simulink model "testBallLQG"  (R2019b)
settings: Solver=VariableStepAuto  StartTime=0.0  StopTime=10.0  RelTol=1e-3
values from neighbouring files (symbols this model uses):
  Ab = [0 1 0 0; 0 0 0 0; 0 0 0 1; 0 0 0 0]    [init.m]    (also in init2.m)
  ballLQRgain = lqr(ballSystem, Q, R)    [init.m]
  ballPosInit = [0.1;0;0;0]    [init.m]    (also in init2.m = [0;0;0;0])
  Bb = [0 0; -g/(1+I_b/(m_b*r_b^2)) 0; 0 0; 0 g/(1+I_b/(m_b*r_b^2))]    [init.m]    (also in init2.m = [0 0; -g/(1+I_b/(m_b*r_b^2) 0; 0 0; 0 g/(1+I_b/(m_b*r_b^2)))
  Cb = [1 0 0 0; 0 0 1 0]    [init.m]    (also in init2.m = [1 0 1 0])
undefined symbols (not defined in the file or in its folder): Continuous, Time
libraries: ctrlSharedLib x1
settings Model: Creator=chukh  LastModifiedBy=chukh

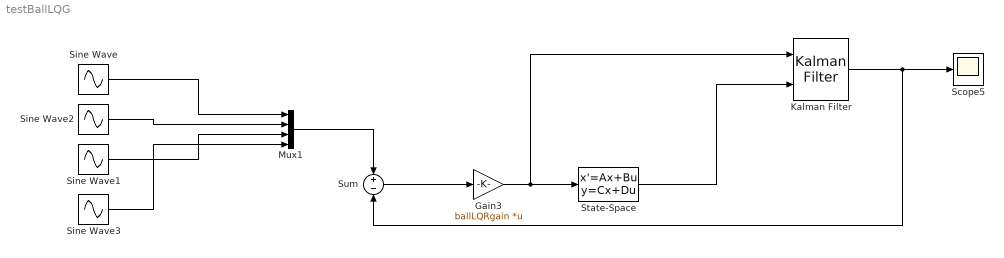
== system testBallLQG ==
  Gain3 : Gain  Gain=ballLQRgain  Multiplication=Matrix(K*u)
  Kalman Filter : ctrlSharedLib/Kalman Filter  TimeDomain=Continuous-Time  UseCurrentEstimator=on  ModelSource=LTI State-Space Variable  ModelSourceVariable=ballSystem  A=0.95  B=1  C=1  D=0  NumberOfStates=1  NumberOfInputs=1  NumberOfOutputs=1  InitialEstimateSource=Dialog  X0=ballPosInit  P0=10  UseK=off  UseGH=off  NumberOfProcessNoiseInputs=1  G=1  TimeInvariantG=on  H=0  TimeInvariantH=on  Q=0.05  TimeInvariantQ=on  R=1  TimeInvariantR=on  N=0  TimeInvariantN=on  AddInputPort=on  AddEnablePort=off  OutputEstimatedY=off  OutputP=off  Ts=-1
      settings: SourceProductBaseCode=CT
  Mux1 : Mux
  Scope5 : Scope
  Sine Wave : Sin  Amplitude=0.1  Phase=pi/2  SampleTime=0
  Sine Wave1 : Sin  Amplitude=0.1  SampleTime=0
  Sine Wave2 : Sin  Amplitude=0.1  Phase=pi  SampleTime=0
  Sine Wave3 : Sin  Amplitude=0.1  Phase=pi/2  SampleTime=0
  State-Space : StateSpace  A=Ab  B=Bb  C=Cb  D=zeros(2,2)  InitialCondition=ballPosInit
  Sum : Sum  Inputs=+-
  wires:
  State-Space/1 -> Kalman Filter/2
  Gain3/1 -> Kalman Filter/1, State-Space/1
  Kalman Filter/1 -> Sum/2, Scope5/1
  Sine Wave1/1 -> Mux1/3
  Sine Wave/1 -> Mux1/1
  Sine Wave2/1 -> Mux1/2
  Sine Wave3/1 -> Mux1/4
  Mux1/1 -> Sum/1
  Sum/1 -> Gain3/1
